simulink model "NonlinearForceControl"  (R2025b)
settings: Solver=VariableStepAuto  StartTime=0.0  StopTime=10  RelTol=1e-3
libraries: roblocks x1, matrix_library x1
settings Model: Creator=Jaxba  LastModifiedBy=Jaxba

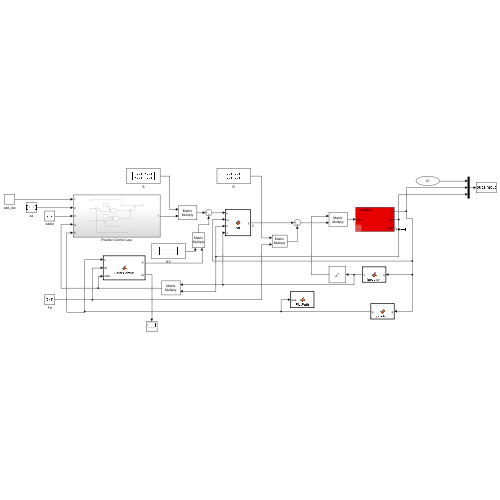
[thumbnail: Simulink's stored preview of the top-level diagram]
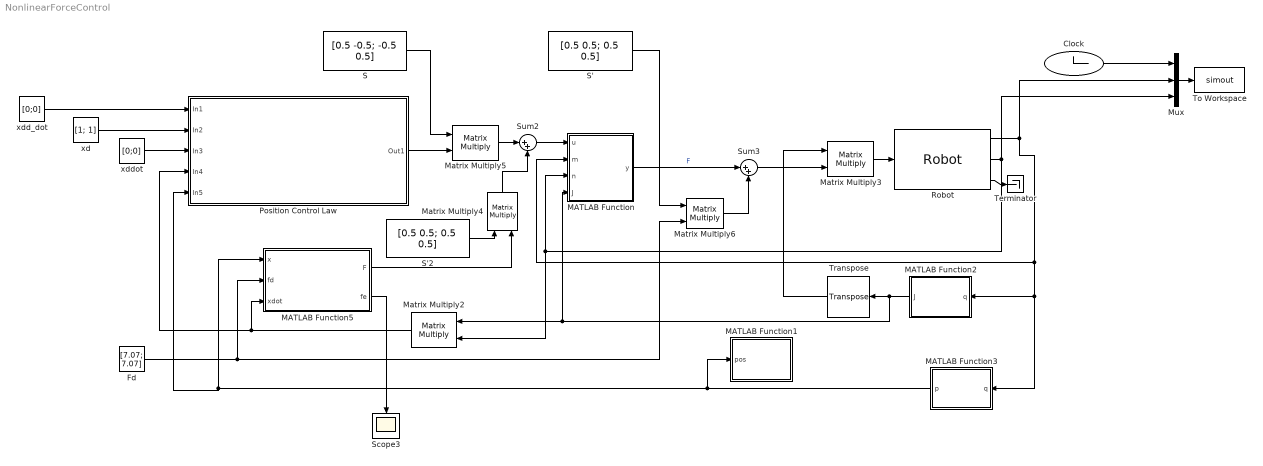
== system NonlinearForceControl ==
  Clock : Clock
  Fd : Constant  Value=[7.07; 7.07]
  MATLAB Function : MATLAB Function  TreatAsAtomicUnit=on
  MATLAB Function1 : MATLAB Function  TreatAsAtomicUnit=on
  MATLAB Function2 : MATLAB Function  TreatAsAtomicUnit=on
  MATLAB Function3 : MATLAB Function  TreatAsAtomicUnit=on
  MATLAB Function5 : MATLAB Function  TreatAsAtomicUnit=on
  Matrix Multiply{2..6} (5 alike) : Product  Multiplication=Matrix(*)
  Mux : Mux  Inputs=3
  Position Control Law : Subsystem
  Robot : roblocks/Robot  robot=SCURRbot  q0=[0 pi/2]
      link override Integrator1: InitialCondition=q0
  S : Constant  Value=[0.5 -0.5; -0.5 0.5]
  S' : Constant  Value=[0.5 0.5; 0.5 0.5]
  S'2 : Constant  Value=[0.5 0.5; 0.5 0.5]
  Scope3 : Scope
      settings: ActiveDisplayYMinimum=-9.1075921608904178  ActiveDisplayYMaximum=81.968329448013776  DataLoggingVariableName=ScopeData3
  Sum2 : Sum  Inputs=|++
  Sum3 : Sum  Inputs=|++
  Terminator : Terminator
  To Workspace : ToWorkspace  VariableName=simout  SampleTime=-1
  Transpose : matrix_library/Transpose
  xd : Constant  Value=[1; 1]
  xdd_dot : Constant  Value=[0;0]
  xddot : Constant  Value=[0;0]
  wires:
  Matrix Multiply3/1 -> Robot/1
  Robot/1 -> Mux/2, MATLAB Function3/1(q), MATLAB Function2/1(q), MATLAB Function/2(m)
  Robot/3 -> Terminator/1
  Matrix Multiply2/1 -> Position Control Law/4(In4), MATLAB Function5/3(xdot)
  Robot/2 -> Mux/3, Matrix Multiply2/2, MATLAB Function/3(n)
  Mux/1 -> To Workspace/1
  Transpose/1 -> Matrix Multiply3/1
  Clock/1 -> Mux/1
  MATLAB Function2/1(J) -> Transpose/1, MATLAB Function/4(J), Matrix Multiply2/1
  Fd/1 -> Matrix Multiply6/2, MATLAB Function5/2(fd)
  S'/1 -> Matrix Multiply6/1
  Sum2/1 -> MATLAB Function/1(u)
  MATLAB Function5/1(F) -> Matrix Multiply4/2
  S'2/1 -> Matrix Multiply4/1
  Matrix Multiply4/1 -> Sum2/2
  MATLAB Function3/1(p) -> Position Control Law/5(In5), MATLAB Function5/1(x), MATLAB Function1/1(pos)
  S/1 -> Matrix Multiply5/1
  Matrix Multiply5/1 -> Sum2/1
  Matrix Multiply6/1 -> Sum3/2
  MATLAB Function/1(y) -> Sum3/1  "F"
  Sum3/1 -> Matrix Multiply3/2
  MATLAB Function5/2(fe) -> Scope3/1
  xdd_dot/1 -> Position Control Law/1(In1)
  xd/1 -> Position Control Law/2(In2)
  xddot/1 -> Position Control Law/3(In3)
  Position Control Law/1(Out1) -> Matrix Multiply5/2

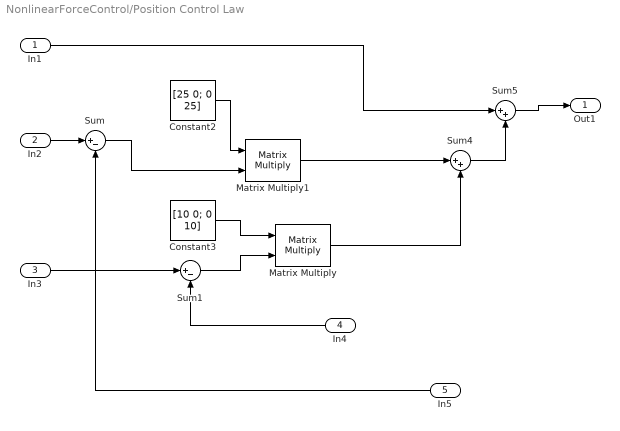
== system NonlinearForceControl/Position Control Law ==
  In1 : Inport
  In2 : Inport  Port=2
  In3 : Inport  Port=3
  In4 : Inport  Port=4
  In5 : Inport  Port=5
  Constant2 : Constant  Value=[25 0; 0 25]
  Constant3 : Constant  Value=[10 0; 0 10]
  Matrix Multiply : Product  Multiplication=Matrix(*)
  Matrix Multiply1 : Product  Multiplication=Matrix(*)
  Sum : Sum  Inputs=|+-
  Sum1 : Sum  Inputs=|+-
  Sum4 : Sum  Inputs=|++
  Sum5 : Sum  Inputs=|++
  Out1 : Outport
  wires:
  Sum4/1 -> Sum5/2
  Sum1/1 -> Matrix Multiply/2
  In4/1 -> Sum1/2
  Sum/1 -> Matrix Multiply1/2
  Constant3/1 -> Matrix Multiply/1
  Matrix Multiply/1 -> Sum4/2
  Matrix Multiply1/1 -> Sum4/1
  In3/1 -> Sum1/1
  Constant2/1 -> Matrix Multiply1/1
  Sum5/1 -> Out1/1
  In1/1 -> Sum5/1
  In2/1 -> Sum/1
  In5/1 -> Sum/2

== matlab function NonlinearForceControl/MATLAB Function1 ==
  data: pos input
function PlotPath(pos)

persistent hFig hAx hTrail hForceArrow initialized

if isempty(initialized)
    % Create figure on first call
    hFig = figure(1001); clf;
    hAx = axes('Parent', hFig);
    hold(hAx, 'on'); grid(hAx, 'on');
    axis(hAx, [-2 2 -2 2]);
    xlabel(hAx, 'X'); ylabel(hAx, 'Y');
    title(hAx, 'End-Effector Path + Wall');

    % --- Add green line y = -x + 2 ---
    xLine = linspace(-2, 2, 200);
    yLine = -xLine + 2;
    plot(hAx, xLine, yLine, 'g-', 'LineWidth', 1.5);

    % Blue path trace
    hTrail = plot(hAx, pos(1), pos(2), 'b.-', 'LineWidth', 2);

    % Placeholder for force arrow
    hForceArrow = quiver(hAx, pos(1), pos(2), 0, 0, 'r', ...
                         'LineWidth', 2, 'MaxHeadSize', 2);

    initialized = true;
end

%% --- Update trail ---
xdata = get(hTrail, 'XData');
ydata = get(hTrail, 'YData');

set(hTrail, 'XData', [xdata pos(1)], ...
            'YData', [ydata pos(2)]);

drawnow limitrate
end

== matlab function NonlinearForceControl/MATLAB Function ==
  data: u input; y output; m input; n input; J input
function y  = fcn(u, m, n, J)

m1 = 3; m2 = 3; B1 = 3; B2 = 3;

m11 = m2+2*m2*cos(m(2))+(m1+m2);
m12 = m2+m2*cos(m(2));
m21 = m2+m2*cos(m(2));
m22 = m2;
M = [m11 m12; m21 m22];

V = [-m2*sin(m(2))*(n(2)^2) - 2*m2*sin(m(2))*n(1)*n(2); 
     m2*sin(m(2))*(n(1)^2)];

F = [B1*n(1); B2*n(2)];

Jinv = inv(J);
JinvT = Jinv';

Jdot11 = -cos(m(1))*n(1) - cos(m(1)+m(2))*(n(1)+n(2));
Jdot12 = -cos(m(1)+m(2)) * (n(1)+n(2));

Jdot21 = -sin(m(1))*n(1) - sin(m(1)+m(2)) * (n(1)+n(2));
Jdot22 = -sin(m(1)+m(2)) * (n(1)+n(2));

Jdot = [Jdot11 Jdot12;
        Jdot21 Jdot22];

Mx = JinvT * M * Jinv;

Vx = JinvT * ( V - (M * Jinv * Jdot * n) );

Fx = JinvT * F;


y = Mx*u + Vx + Fx;
end

== matlab function NonlinearForceControl/MATLAB Function2 ==
  data: q input; J output
function J = jacobian(q)

% Jacobian for 2R arm
J11 = -sin(q(1)) - sin(q(1)+q(2));
J12 = -sin(q(1)+q(2));

J21 =  cos(q(1)) + cos(q(1)+q(2));
J22 =  cos(q(1)+q(2));

J = [J11 J12;
     J21 J22];
end

== matlab function NonlinearForceControl/MATLAB Function3 ==
  data: q input; p output
function p = position(q)

% Forward kinematics
x = cos(q(1)) + cos(q(1) + q(2));
y = sin(q(1)) + sin(q(1) + q(2));

p = [x; y];
end

== matlab function NonlinearForceControl/MATLAB Function5 ==
  data: x input; fd input; xdot input; F output; fe output
function [F, fe]= ForceControl(x, fd, xdot)
   
    Kenv = 1000;
    Kpf  = 25;
    Kvf  = 10;

    n = [1;1]/sqrt(2);      % Direction of force normal
    d = n' * x - 2/sqrt(2); % Distance into wall
    

    if d < 0
        fe = [0; 0];
    else
        fe = Kenv*d*n;
    end

    ef = fd - fe;

    xdot_n = n' * xdot;      % scalar velocity along normal
    xdot_proj = xdot_n * n;  % vector velocity along normal

    F = (Kpf/Kenv)*ef - Kvf*xdot_proj;
end
